simulink model "sampleModel2432_pp"  (R2018a)
settings: Solver=VariableStepAuto  StartTime=0.0  StopTime=10.0  RelTol=1e-3
undefined symbols (not defined in the file or in its folder): DiscIntNeverNeededParam, sigbuilder_block
libraries: simulink x354
(part 4 of 8)

== system sampleModel2432_pp/cfblk235 ==
  cfblk1 : Inport
  Action Port : ActionPort  ActionType=then
  cfblk10 : Delay
  cfblk3 : Delay  ShowEnablePort=on
      settings: InputPortMap=u0,e6
  cfblk4 : DiscreteIntegrator  SampleTime=-1  ICPrevOutput=DiscIntNeverNeededParam  ICPrevScaledInput=DiscIntNeverNeededParam
  cfblk5 : simulink/Continuous/PID Controller  Controller=PID  TimeDomain=Discrete-time  SampleTime=-1  IntegratorMethod=Forward Euler  FilterMethod=Forward Euler  Form=Parallel  UseFilter=on  ControllerParametersSource=internal  P=1  I=1  D=0  N=100  InitialConditionSource=internal  InitialConditionForIntegrator=0  InitialConditionForFilter=0  ExternalReset=none  LimitOutput=off  UpperSaturationLimit=inf  LowerSaturationLimit=-inf  LinearizeAsGain=off  AntiWindupMode=none  Kb=1  TrackingMode=off  Kt=1  PParamMin=[]  PParamMax=[]  IParamMin=[]  IParamMax=[]  DParamMin=[]  DParamMax=[]  NParamMin=[]  NParamMax=[]  KbParamMin=[]  KbParamMax=[]  KtParamMin=[]  KtParamMax=[]  POutMin=[]  POutMax=[]  IOutMin=[]  IOutMax=[]  DOutMin=[]  DOutMax=[]  NOutMin=[]  NOutMax=[]  KbOutMin=[]  KbOutMax=[]  KtOutMin=[]  KtOutMax=[]  IntegratorOutMin=[]  IntegratorOutMax=[]  FilterOutMin=[]  FilterOutMax=[]  SumOutMin=[]  SumOutMax=[]  SumI1OutMin=[]  SumI1OutMax=[]  SumI2OutMin=[]  SumI2OutMax=[]  SumI3OutMin=[]  SumI3OutMax=[]  SumDOutMin=[]  SumDOutMax=[]  SaturationOutMin=[]  SaturationOutMax=[]  IntegratorContinuousStateAttributes=''  IntegratorStateMustResolveToSignalObject=off  IntegratorRTWStateStorageClass=Auto  FilterContinuousStateAttributes=''  FilterStateMustResolveToSignalObject=off  FilterRTWStateStorageClass=Auto  DifferentiatorICPrevScaledInput=0  DifferentiatorOutMin=[]  DifferentiatorOutMax=[]  FilterDiffOutCoefMin=[]  FilterDiffOutCoefMax=[]  SumDenOutMin=[]  SumDenOutMax=[]  SumNumOutMin=[]  SumNumOutMax=[]  ReciprocalOutMin=[]  ReciprocalOutMax=[]  DivideOutMin=[]  DivideOutMax=[]  TunerSelectOption=Transfer Function Based (PID Tuner App)
  cfblk6 : Delay  ShowEnablePort=on
      settings: InputPortMap=u0,e6
  cfblk7 : Delay
  cfblk9 : Delay
  cyemi_{926..934} (9 alike) : DataTypeConversion  OutDataTypeStr=double
  cfblk2 : Outport
  cfblk8 : Outport  Port=2
  wires:
  cfblk1/1 -> cfblk2/1, cyemi_931/1
  cfblk7/1 -> cfblk8/1, cyemi_926/1, cyemi_932/1
  cyemi_926/1 -> cfblk10/1
  cyemi_927/1 -> cfblk3/1
  cfblk9/1 -> cyemi_927/1
  cyemi_928/1 -> cfblk3/2
  cfblk6/1 -> cyemi_928/1
  cyemi_929/1 -> cfblk4/1
  cfblk10/1 -> cyemi_929/1
  cyemi_930/1 -> cfblk5/1
  cfblk3/1 -> cyemi_930/1
  cyemi_931/1 -> cfblk6/1
  cyemi_932/1 -> cfblk6/2
  cyemi_933/1 -> cfblk7/1
  cfblk4/1 -> cyemi_933/1
  cyemi_934/1 -> cfblk9/1
  cfblk5/1 -> cyemi_934/1

== system sampleModel2432_pp/cfblk236 ==
  cfblk1 : Inport
  Action Port : ActionPort  ActionType=else
  cfblk{9..12} (4 alike) : DiscreteIntegrator  SampleTime=-1  ICPrevOutput=DiscIntNeverNeededParam  ICPrevScaledInput=DiscIntNeverNeededParam
  cfblk13 : simulink/Discrete/Transfer Fcn First Order  PoleZ=0.95  ICPrevOutput=0.0  DoSatur=off
      settings: SourceProductName=Simulink
  cfblk3 : simulink/Continuous/PID Controller  Controller=PID  TimeDomain=Discrete-time  SampleTime=-1  IntegratorMethod=Forward Euler  FilterMethod=Forward Euler  Form=Parallel  UseFilter=on  ControllerParametersSource=internal  P=1  I=1  D=0  N=100  InitialConditionSource=internal  InitialConditionForIntegrator=0  InitialConditionForFilter=0  ExternalReset=none  LimitOutput=off  UpperSaturationLimit=inf  LowerSaturationLimit=-inf  LinearizeAsGain=off  AntiWindupMode=none  Kb=1  TrackingMode=off  Kt=1  PParamMin=[]  PParamMax=[]  IParamMin=[]  IParamMax=[]  DParamMin=[]  DParamMax=[]  NParamMin=[]  NParamMax=[]  KbParamMin=[]  KbParamMax=[]  KtParamMin=[]  KtParamMax=[]  POutMin=[]  POutMax=[]  IOutMin=[]  IOutMax=[]  DOutMin=[]  DOutMax=[]  NOutMin=[]  NOutMax=[]  KbOutMin=[]  KbOutMax=[]  KtOutMin=[]  KtOutMax=[]  IntegratorOutMin=[]  IntegratorOutMax=[]  FilterOutMin=[]  FilterOutMax=[]  SumOutMin=[]  SumOutMax=[]  SumI1OutMin=[]  SumI1OutMax=[]  SumI2OutMin=[]  SumI2OutMax=[]  SumI3OutMin=[]  SumI3OutMax=[]  SumDOutMin=[]  SumDOutMax=[]  SaturationOutMin=[]  SaturationOutMax=[]  IntegratorContinuousStateAttributes=''  IntegratorStateMustResolveToSignalObject=off  IntegratorRTWStateStorageClass=Auto  FilterContinuousStateAttributes=''  FilterStateMustResolveToSignalObject=off  FilterRTWStateStorageClass=Auto  DifferentiatorICPrevScaledInput=0  DifferentiatorOutMin=[]  DifferentiatorOutMax=[]  FilterDiffOutCoefMin=[]  FilterDiffOutCoefMax=[]  SumDenOutMin=[]  SumDenOutMax=[]  SumNumOutMin=[]  SumNumOutMax=[]  ReciprocalOutMin=[]  ReciprocalOutMax=[]  DivideOutMin=[]  DivideOutMax=[]  TunerSelectOption=Transfer Function Based (PID Tuner App)
  cfblk4 : simulink/Discrete/Tapped Delay  vinit=0.0  samptime=-1  NumDelays=1  DelayOrder=Oldest  includeCurrent=off
  cfblk5 : Delay  DelayLengthSource=Input port
      settings: InputPortMap=u0,p1
  cfblk6 : Delay  ShowEnablePort=on
      settings: InputPortMap=u0,e6
  cfblk7 : Delay
  cfblk8 : DiscreteTransferFcn
  cyemi_{936..948} (13 alike) : DataTypeConversion  OutDataTypeStr=double
  cfblk2 : Outport
  wires:
  cfblk3/1 -> cyemi_939/1, cyemi_941/1
  cfblk1/1 -> cyemi_940/1, cyemi_945/1
  cfblk5/1 -> cfblk2/1
  cyemi_936/1 -> cfblk10/1
  cfblk8/1 -> cyemi_936/1
  cyemi_937/1 -> cfblk11/1
  cfblk12/1 -> cyemi_937/1
  cyemi_938/1 -> cfblk12/1
  cfblk10/1 -> cyemi_938/1
  cyemi_939/1 -> cfblk13/1
  cyemi_940/1 -> cfblk3/1
  cyemi_941/1 -> cfblk4/1
  cyemi_942/1 -> cfblk5/1
  cfblk7/1 -> cyemi_942/1
  cyemi_943/1 -> cfblk5/2
  cfblk11/1 -> cyemi_943/1
  cyemi_944/1 -> cfblk6/1
  cfblk4/1 -> cyemi_944/1
  cyemi_945/1 -> cfblk6/2
  cyemi_946/1 -> cfblk7/1
  cfblk6/1 -> cyemi_946/1
  cyemi_947/1 -> cfblk8/1
  cfblk9/1 -> cyemi_947/1
  cyemi_948/1 -> cfblk9/1
  cfblk13/1 -> cyemi_948/1

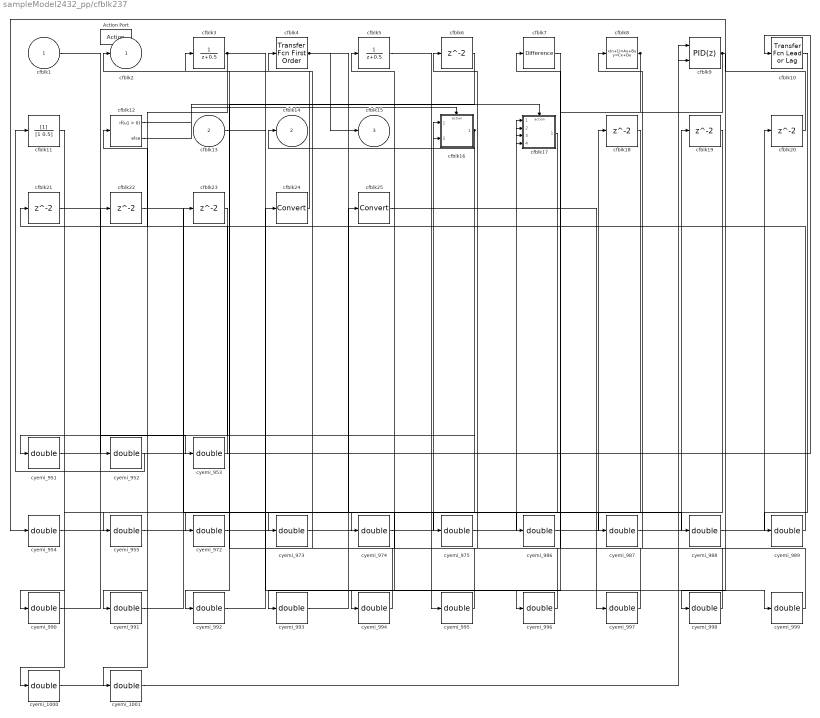
== system sampleModel2432_pp/cfblk237 ==
  cfblk1 : Inport
  cfblk13 : Inport  Port=2
  Action Port : ActionPort  ActionType=then
  cfblk10 : simulink/Discrete/Transfer Fcn Lead or Lag  PoleZ=0.95  ZeroZ=0.75  ICPrevOutput=0.0  ICPrevInput=0.0  DoSatur=off
      settings: SourceProductName=Simulink  SourceProductBaseCode=SL
  cfblk11 : DiscreteFilter
  cfblk12 : If  SampleTime=1
  cfblk16 : Subsystem  TreatAsAtomicUnit=on
  cfblk17 : Subsystem  TreatAsAtomicUnit=on
  cfblk{6,18..23} (7 alike) : Delay
  cfblk24 : DataTypeConversion
  cfblk25 : DataTypeConversion
  cfblk3 : DiscreteTransferFcn
  cfblk4 : simulink/Discrete/Transfer Fcn First Order  PoleZ=0.95  ICPrevOutput=0.0  DoSatur=off
      settings: SourceProductName=Simulink
  cfblk5 : DiscreteTransferFcn
  cfblk7 : simulink/Discrete/Difference  ICPrevInput=0.0  OutMin=[]  OutMax=[]  OutDataTypeStr=Inherit: Inherit via back propagation  OutDataType=fixdt(1, 16)  OutScaling=2^-10  DoSatur=off
  cfblk8 : DiscreteStateSpace  SampleTime=-1
  cfblk9 : simulink/Continuous/PID Controller (2DOF)  Controller=PID  TimeDomain=Discrete-time  SampleTime=-1  IntegratorMethod=Forward Euler  FilterMethod=Forward Euler  Form=Parallel  UseFilter=on  ControllerParametersSource=internal  P=1  I=1  D=0  N=100  b=1  c=1  InitialConditionSource=internal  InitialConditionForIntegrator=0  InitialConditionForFilter=0  ExternalReset=none  LimitOutput=off  UpperSaturationLimit=inf  LowerSaturationLimit=-inf  LinearizeAsGain=off  AntiWindupMode=none  Kb=1  TrackingMode=off  Kt=1  PParamMin=[]  PParamMax=[]  IParamMin=[]  IParamMax=[]  DParamMin=[]  DParamMax=[]  NParamMin=[]  NParamMax=[]  bParamMin=[]  bParamMax=[]  cParamMin=[]  cParamMax=[]  KbParamMin=[]  KbParamMax=[]  KtParamMin=[]  KtParamMax=[]  POutMin=[]  POutMax=[]  IOutMin=[]  IOutMax=[]  DOutMin=[]  DOutMax=[]  NOutMin=[]  NOutMax=[]  bOutMin=[]  bOutMax=[]  cOutMin=[]  cOutMax=[]  KbOutMin=[]  KbOutMax=[]  KtOutMin=[]  KtOutMax=[]  IntegratorOutMin=[]  IntegratorOutMax=[]  FilterOutMin=[]  FilterOutMax=[]  SumOutMin=[]  SumOutMax=[]  Sum1OutMin=[]  Sum1OutMax=[]  Sum2OutMin=[]  Sum2OutMax=[]  Sum3OutMin=[]  Sum3OutMax=[]  SumI1OutMin=[]  SumI1OutMax=[]  SumI2OutMin=[]  SumI2OutMax=[]  SumI3OutMin=[]  SumI3OutMax=[]  SumDOutMin=[]  SumDOutMax=[]  SaturationOutMin=[]  SaturationOutMax=[]  IntegratorContinuousStateAttributes=''  IntegratorStateMustResolveToSignalObject=off  IntegratorRTWStateStorageClass=Auto  FilterContinuousStateAttributes=''  FilterStateMustResolveToSignalObject=off  FilterRTWStateStorageClass=Auto  DifferentiatorICPrevScaledInput=0  DifferentiatorOutMin=[]  DifferentiatorOutMax=[]  FilterDiffOutCoefMin=[]  FilterDiffOutCoefMax=[]  SumDenOutMin=[]  SumDenOutMax=[]  SumNumOutMin=[]  SumNumOutMax=[]  ReciprocalOutMin=[]  ReciprocalOutMax=[]  DivideOutMin=[]  DivideOutMax=[]  TunerSelectOption=Transfer Function Based (PID Tuner App)
  cyemi_{951..955,972..975,986..1001} (25 alike) : DataTypeConversion  OutDataTypeStr=double
  cfblk2 : Outport
  cfblk14 : Outport  Port=2
  cfblk15 : Outport  Port=3
  wires:
  cfblk4/1 -> cfblk15/1, cyemi_986/1
  cfblk16/1(cfblk2) -> cfblk14/1, cyemi_951/1, cyemi_990/1
  cfblk8/1 -> cyemi_973/1, cyemi_993/1
  cfblk9/1 -> cyemi_975/1, cyemi_998/1
  cfblk3/1 -> cyemi_987/1, cyemi_988/1, cyemi_991/1
  cfblk12/1 -> cfblk16/Action
  cfblk12/2 -> cfblk17/Action
  cfblk24/1 -> cfblk2/1
  cyemi_951/1 -> cfblk10/1
  cyemi_952/1 -> cfblk11/1
  cfblk1/1 -> cyemi_952/1
  cyemi_953/1 -> cfblk12/1
  cfblk21/1 -> cyemi_953/1
  cyemi_954/1 -> cfblk16/1(cfblk1)
  cfblk20/1 -> cyemi_954/1
  cyemi_955/1 -> cfblk16/2(cfblk16)
  cfblk23/1 -> cyemi_955/1
  cyemi_972/1 -> cfblk17/1(cfblk1)
  cfblk19/1 -> cyemi_972/1
  cyemi_973/1 -> cfblk17/2(cfblk10)
  cyemi_974/1 -> cfblk17/3(cfblk11)
  cfblk22/1 -> cyemi_974/1
  cyemi_975/1 -> cfblk17/4(cfblk12)
  cyemi_986/1 -> cfblk18/1
  cyemi_987/1 -> cfblk19/1
  cyemi_988/1 -> cfblk20/1
  cyemi_989/1 -> cfblk21/1
  cfblk10/1 -> cyemi_989/1
  cyemi_990/1 -> cfblk22/1
  cyemi_991/1 -> cfblk23/1
  cyemi_992/1 -> cfblk24/1
  cfblk6/1 -> cyemi_992/1
  cyemi_993/1 -> cfblk25/1
  cyemi_994/1 -> cfblk3/1
  cfblk17/1(cfblk2) -> cyemi_994/1
  cyemi_995/1 -> cfblk4/1
  cfblk5/1 -> cyemi_995/1
  cyemi_996/1 -> cfblk5/1
  cfblk7/1 -> cyemi_996/1
  cyemi_997/1 -> cfblk6/1
  cfblk25/1 -> cyemi_997/1
  cyemi_998/1 -> cfblk7/1
  cyemi_999/1 -> cfblk8/1
  cfblk13/1 -> cyemi_999/1
  cyemi_1000/1 -> cfblk9/1
  cfblk11/1 -> cyemi_1000/1
  cyemi_1001/1 -> cfblk9/2
  cfblk18/1 -> cyemi_1001/1

== system sampleModel2432_pp/cfblk238 ==
  cfblk1 : Inport
  cfblk12 : Inport  Port=2
  Action Port : ActionPort  ActionType=else
  cfblk10 : DiscreteIntegrator  SampleTime=-1  ICPrevOutput=DiscIntNeverNeededParam  ICPrevScaledInput=DiscIntNeverNeededParam
  cfblk11 : Delay  ShowEnablePort=on
      settings: InputPortMap=u0,e6
  cfblk16 : Delay
  cfblk17 : Delay
  cfblk3 : DiscreteFilter
  cfblk4 : simulink/Discrete/Difference  ICPrevInput=0.0  OutMin=[]  OutMax=[]  OutDataTypeStr=Inherit: Inherit via back propagation  OutDataType=fixdt(1, 16)  OutScaling=2^-10  DoSatur=off
  cfblk5 : simulink/Continuous/PID Controller  Controller=PID  TimeDomain=Discrete-time  SampleTime=-1  IntegratorMethod=Forward Euler  FilterMethod=Forward Euler  Form=Parallel  UseFilter=on  ControllerParametersSource=internal  P=1  I=1  D=0  N=100  InitialConditionSource=internal  InitialConditionForIntegrator=0  InitialConditionForFilter=0  ExternalReset=none  LimitOutput=off  UpperSaturationLimit=inf  LowerSaturationLimit=-inf  LinearizeAsGain=off  AntiWindupMode=none  Kb=1  TrackingMode=off  Kt=1  PParamMin=[]  PParamMax=[]  IParamMin=[]  IParamMax=[]  DParamMin=[]  DParamMax=[]  NParamMin=[]  NParamMax=[]  KbParamMin=[]  KbParamMax=[]  KtParamMin=[]  KtParamMax=[]  POutMin=[]  POutMax=[]  IOutMin=[]  IOutMax=[]  DOutMin=[]  DOutMax=[]  NOutMin=[]  NOutMax=[]  KbOutMin=[]  KbOutMax=[]  KtOutMin=[]  KtOutMax=[]  IntegratorOutMin=[]  IntegratorOutMax=[]  FilterOutMin=[]  FilterOutMax=[]  SumOutMin=[]  SumOutMax=[]  SumI1OutMin=[]  SumI1OutMax=[]  SumI2OutMin=[]  SumI2OutMax=[]  SumI3OutMin=[]  SumI3OutMax=[]  SumDOutMin=[]  SumDOutMax=[]  SaturationOutMin=[]  SaturationOutMax=[]  IntegratorContinuousStateAttributes=''  IntegratorStateMustResolveToSignalObject=off  IntegratorRTWStateStorageClass=Auto  FilterContinuousStateAttributes=''  FilterStateMustResolveToSignalObject=off  FilterRTWStateStorageClass=Auto  DifferentiatorICPrevScaledInput=0  DifferentiatorOutMin=[]  DifferentiatorOutMax=[]  FilterDiffOutCoefMin=[]  FilterDiffOutCoefMax=[]  SumDenOutMin=[]  SumDenOutMax=[]  SumNumOutMin=[]  SumNumOutMax=[]  ReciprocalOutMin=[]  ReciprocalOutMax=[]  DivideOutMin=[]  DivideOutMax=[]  TunerSelectOption=Transfer Function Based (PID Tuner App)
  cfblk6 : simulink/Continuous/PID Controller (2DOF)  Controller=PID  TimeDomain=Discrete-time  SampleTime=-1  IntegratorMethod=Forward Euler  FilterMethod=Forward Euler  Form=Parallel  UseFilter=on  ControllerParametersSource=internal  P=1  I=1  D=0  N=100  b=1  c=1  InitialConditionSource=internal  InitialConditionForIntegrator=0  InitialConditionForFilter=0  ExternalReset=none  LimitOutput=off  UpperSaturationLimit=inf  LowerSaturationLimit=-inf  LinearizeAsGain=off  AntiWindupMode=none  Kb=1  TrackingMode=off  Kt=1  PParamMin=[]  PParamMax=[]  IParamMin=[]  IParamMax=[]  DParamMin=[]  DParamMax=[]  NParamMin=[]  NParamMax=[]  bParamMin=[]  bParamMax=[]  cParamMin=[]  cParamMax=[]  KbParamMin=[]  KbParamMax=[]  KtParamMin=[]  KtParamMax=[]  POutMin=[]  POutMax=[]  IOutMin=[]  IOutMax=[]  DOutMin=[]  DOutMax=[]  NOutMin=[]  NOutMax=[]  bOutMin=[]  bOutMax=[]  cOutMin=[]  cOutMax=[]  KbOutMin=[]  KbOutMax=[]  KtOutMin=[]  KtOutMax=[]  IntegratorOutMin=[]  IntegratorOutMax=[]  FilterOutMin=[]  FilterOutMax=[]  SumOutMin=[]  SumOutMax=[]  Sum1OutMin=[]  Sum1OutMax=[]  Sum2OutMin=[]  Sum2OutMax=[]  Sum3OutMin=[]  Sum3OutMax=[]  SumI1OutMin=[]  SumI1OutMax=[]  SumI2OutMin=[]  SumI2OutMax=[]  SumI3OutMin=[]  SumI3OutMax=[]  SumDOutMin=[]  SumDOutMax=[]  SaturationOutMin=[]  SaturationOutMax=[]  IntegratorContinuousStateAttributes=''  IntegratorStateMustResolveToSignalObject=off  IntegratorRTWStateStorageClass=Auto  FilterContinuousStateAttributes=''  FilterStateMustResolveToSignalObject=off  FilterRTWStateStorageClass=Auto  DifferentiatorICPrevScaledInput=0  DifferentiatorOutMin=[]  DifferentiatorOutMax=[]  FilterDiffOutCoefMin=[]  FilterDiffOutCoefMax=[]  SumDenOutMin=[]  SumDenOutMax=[]  SumNumOutMin=[]  SumNumOutMax=[]  ReciprocalOutMin=[]  ReciprocalOutMax=[]  DivideOutMin=[]  DivideOutMax=[]  TunerSelectOption=Transfer Function Based (PID Tuner App)
  cfblk7 : simulink/Discrete/Transfer Fcn First Order  PoleZ=0.95  ICPrevOutput=0.0  DoSatur=off
      settings: SourceProductName=Simulink
  cfblk8 : simulink/Discrete/Transfer Fcn First Order  PoleZ=0.95  ICPrevOutput=0.0  DoSatur=off
      settings: SourceProductName=Simulink
  cfblk9 : UnitDelay  SampleTime=-1
  cyemi_{1004..1016} (13 alike) : DataTypeConversion  OutDataTypeStr=double
  cfblk2 : Outport
  cfblk13 : Outport  Port=2
  cfblk14 : Outport  Port=3
  cfblk15 : Outport  Port=4
  wires:
  cfblk6/1 -> cfblk15/1, cyemi_1007/1
  cfblk9/1 -> cfblk14/1
  cfblk11/1 -> cyemi_1004/1, cyemi_1013/1, cyemi_1014/1
  cfblk3/1 -> cfblk2/1, cyemi_1010/1
  cfblk12/1 -> cfblk13/1
  cyemi_1004/1 -> cfblk10/1
  cyemi_1005/1 -> cfblk11/1
  cfblk5/1 -> cyemi_1005/1
  cyemi_1006/1 -> cfblk11/2
  cfblk16/1 -> cyemi_1006/1
  cyemi_1007/1 -> cfblk16/1
  cyemi_1008/1 -> cfblk17/1
  cfblk10/1 -> cyemi_1008/1
  cyemi_1009/1 -> cfblk3/1
  cfblk17/1 -> cyemi_1009/1
  cyemi_1010/1 -> cfblk4/1
  cyemi_1011/1 -> cfblk5/1
  cfblk4/1 -> cyemi_1011/1
  cyemi_1012/1 -> cfblk6/1
  cfblk7/1 -> cyemi_1012/1
  cyemi_1013/1 -> cfblk6/2
  cyemi_1014/1 -> cfblk7/1
  cyemi_1015/1 -> cfblk8/1
  cfblk1/1 -> cyemi_1015/1
  cyemi_1016/1 -> cfblk9/1
  cfblk8/1 -> cyemi_1016/1

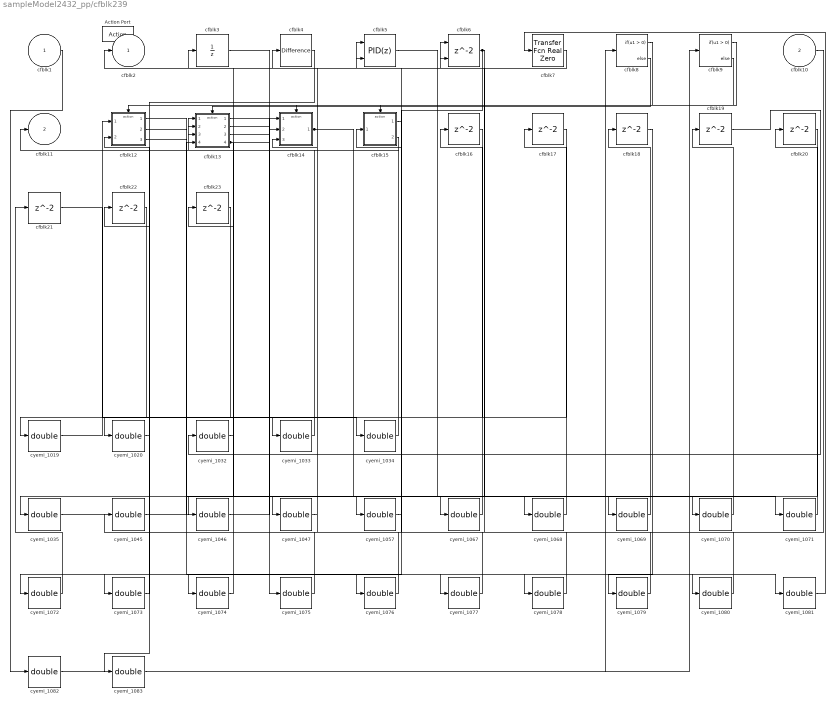
== system sampleModel2432_pp/cfblk239 ==
  cfblk1 : Inport
  cfblk10 : Inport  Port=2
  Action Port : ActionPort  ActionType=then
  cfblk12 : Subsystem  TreatAsAtomicUnit=on
  cfblk13 : Subsystem  TreatAsAtomicUnit=on
  cfblk14 : Subsystem  TreatAsAtomicUnit=on
  cfblk15 : Subsystem  TreatAsAtomicUnit=on
  cfblk{16..23} (8 alike) : Delay
  cfblk3 : UnitDelay  SampleTime=-1
  cfblk4 : simulink/Discrete/Difference  ICPrevInput=0.0  OutMin=[]  OutMax=[]  OutDataTypeStr=Inherit: Inherit via back propagation  OutDataType=fixdt(1, 16)  OutScaling=2^-10  DoSatur=off
  cfblk5 : simulink/Continuous/PID Controller (2DOF)  Controller=PID  TimeDomain=Discrete-time  SampleTime=-1  IntegratorMethod=Forward Euler  FilterMethod=Forward Euler  Form=Parallel  UseFilter=on  ControllerParametersSource=internal  P=1  I=1  D=0  N=100  b=1  c=1  InitialConditionSource=internal  InitialConditionForIntegrator=0  InitialConditionForFilter=0  ExternalReset=none  LimitOutput=off  UpperSaturationLimit=inf  LowerSaturationLimit=-inf  LinearizeAsGain=off  AntiWindupMode=none  Kb=1  TrackingMode=off  Kt=1  PParamMin=[]  PParamMax=[]  IParamMin=[]  IParamMax=[]  DParamMin=[]  DParamMax=[]  NParamMin=[]  NParamMax=[]  bParamMin=[]  bParamMax=[]  cParamMin=[]  cParamMax=[]  KbParamMin=[]  KbParamMax=[]  KtParamMin=[]  KtParamMax=[]  POutMin=[]  POutMax=[]  IOutMin=[]  IOutMax=[]  DOutMin=[]  DOutMax=[]  NOutMin=[]  NOutMax=[]  bOutMin=[]  bOutMax=[]  cOutMin=[]  cOutMax=[]  KbOutMin=[]  KbOutMax=[]  KtOutMin=[]  KtOutMax=[]  IntegratorOutMin=[]  IntegratorOutMax=[]  FilterOutMin=[]  FilterOutMax=[]  SumOutMin=[]  SumOutMax=[]  Sum1OutMin=[]  Sum1OutMax=[]  Sum2OutMin=[]  Sum2OutMax=[]  Sum3OutMin=[]  Sum3OutMax=[]  SumI1OutMin=[]  SumI1OutMax=[]  SumI2OutMin=[]  SumI2OutMax=[]  SumI3OutMin=[]  SumI3OutMax=[]  SumDOutMin=[]  SumDOutMax=[]  SaturationOutMin=[]  SaturationOutMax=[]  IntegratorContinuousStateAttributes=''  IntegratorStateMustResolveToSignalObject=off  IntegratorRTWStateStorageClass=Auto  FilterContinuousStateAttributes=''  FilterStateMustResolveToSignalObject=off  FilterRTWStateStorageClass=Auto  DifferentiatorICPrevScaledInput=0  DifferentiatorOutMin=[]  DifferentiatorOutMax=[]  FilterDiffOutCoefMin=[]  FilterDiffOutCoefMax=[]  SumDenOutMin=[]  SumDenOutMax=[]  SumNumOutMin=[]  SumNumOutMax=[]  ReciprocalOutMin=[]  ReciprocalOutMax=[]  DivideOutMin=[]  DivideOutMax=[]  TunerSelectOption=Transfer Function Based (PID Tuner App)
  cfblk6 : Delay  ShowEnablePort=on
      settings: InputPortMap=u0,e6
  cfblk7 : simulink/Discrete/Transfer Fcn Real Zero  ZeroZ=0.75  ICPrevInput=0.0  DoSatur=off
      settings: SourceProductName=Simulink  SourceProductBaseCode=SL
  cfblk8 : If  SampleTime=1
  cfblk9 : If  SampleTime=1
  cyemi_{1019..1020,1032..1035,1045..1047,1057,1067..1083} (27 alike) : DataTypeConversion  OutDataTypeStr=double
  cfblk2 : Outport
  cfblk11 : Outport  Port=2
  wires:
  cfblk7/1 -> cfblk2/1
  cfblk14/1(cfblk2) -> cyemi_1070/1, cyemi_1071/1
  cfblk15/2(cfblk11) -> cfblk11/1
  cfblk6/1 -> cyemi_1047/1, cyemi_1067/1, cyemi_1072/1
  cfblk13/4(cfblk16) -> cyemi_1046/1, cyemi_1081/1
  cfblk8/1 -> cfblk12/Action
  cfblk8/2 -> cfblk13/Action
  cfblk9/1 -> cfblk14/Action
  cfblk9/2 -> cfblk15/Action
  cyemi_1019/1 -> cfblk12/1(cfblk1)
  cfblk17/1 -> cyemi_1019/1
  cyemi_1020/1 -> cfblk12/2(cfblk12)
  cfblk22/1 -> cyemi_1020/1
  cyemi_1032/1 -> cfblk13/1(cfblk1)
  cfblk19/1 -> cyemi_1032/1
  cyemi_1033/1 -> cfblk13/2(cfblk11)
  cfblk16/1 -> cyemi_1033/1
  cyemi_1034/1 -> cfblk13/3(cfblk12)
  cfblk21/1 -> cyemi_1034/1
  cyemi_1035/1 -> cfblk13/4(cfblk13)
  cfblk20/1 -> cyemi_1035/1
  cyemi_1045/1 -> cfblk14/1(cfblk1)
  cfblk10/1 -> cyemi_1045/1
  cyemi_1046/1 -> cfblk14/2(cfblk12)
  cyemi_1047/1 -> cfblk14/3(cfblk13)
  cyemi_1057/1 -> cfblk15/1(cfblk1)
  cfblk12/3(cfblk14) -> cyemi_1057/1
  cyemi_1067/1 -> cfblk16/1
  cyemi_1068/1 -> cfblk17/1
  cfblk5/1 -> cyemi_1068/1
  cyemi_1069/1 -> cfblk18/1
  cfblk3/1 -> cyemi_1069/1
  cyemi_1070/1 -> cfblk19/1
  cyemi_1071/1 -> cfblk20/1
  cyemi_1072/1 -> cfblk21/1
  cyemi_1073/1 -> cfblk22/1
  cfblk4/1 -> cyemi_1073/1
  cyemi_1074/1 -> cfblk23/1
  cfblk15/1(cfblk2) -> cyemi_1074/1
  cyemi_1075/1 -> cfblk3/1
  cfblk13/3(cfblk15) -> cyemi_1075/1
  cyemi_1076/1 -> cfblk4/1
  cfblk12/2(cfblk13) -> cyemi_1076/1
  cyemi_1077/1 -> cfblk5/1
  cfblk13/1(cfblk2) -> cyemi_1077/1
  cyemi_1078/1 -> cfblk5/2
  cfblk13/2(cfblk14) -> cyemi_1078/1
  cyemi_1079/1 -> cfblk6/1
  cfblk18/1 -> cyemi_1079/1
  cyemi_1080/1 -> cfblk6/2
  cfblk12/1(cfblk2) -> cyemi_1080/1
  cyemi_1081/1 -> cfblk7/1
  cyemi_1082/1 -> cfblk8/1
  cfblk1/1 -> cyemi_1082/1
  cyemi_1083/1 -> cfblk9/1
  cfblk23/1 -> cyemi_1083/1

== system sampleModel2432_pp/cfblk240 ==
  cfblk1 : Inport
  cfblk7 : Inport  Port=2
  Action Port : ActionPort  ActionType=else
  cfblk3 : simulink/Discrete/Tapped Delay  vinit=0.0  samptime=-1  NumDelays=1  DelayOrder=Oldest  includeCurrent=off
  cfblk4 : DiscreteTransferFcn
  cfblk5 : simulink/Continuous/PID Controller  Controller=PID  TimeDomain=Discrete-time  SampleTime=-1  IntegratorMethod=Forward Euler  FilterMethod=Forward Euler  Form=Parallel  UseFilter=on  ControllerParametersSource=internal  P=1  I=1  D=0  N=100  InitialConditionSource=internal  InitialConditionForIntegrator=0  InitialConditionForFilter=0  ExternalReset=none  LimitOutput=off  UpperSaturationLimit=inf  LowerSaturationLimit=-inf  LinearizeAsGain=off  AntiWindupMode=none  Kb=1  TrackingMode=off  Kt=1  PParamMin=[]  PParamMax=[]  IParamMin=[]  IParamMax=[]  DParamMin=[]  DParamMax=[]  NParamMin=[]  NParamMax=[]  KbParamMin=[]  KbParamMax=[]  KtParamMin=[]  KtParamMax=[]  POutMin=[]  POutMax=[]  IOutMin=[]  IOutMax=[]  DOutMin=[]  DOutMax=[]  NOutMin=[]  NOutMax=[]  KbOutMin=[]  KbOutMax=[]  KtOutMin=[]  KtOutMax=[]  IntegratorOutMin=[]  IntegratorOutMax=[]  FilterOutMin=[]  FilterOutMax=[]  SumOutMin=[]  SumOutMax=[]  SumI1OutMin=[]  SumI1OutMax=[]  SumI2OutMin=[]  SumI2OutMax=[]  SumI3OutMin=[]  SumI3OutMax=[]  SumDOutMin=[]  SumDOutMax=[]  SaturationOutMin=[]  SaturationOutMax=[]  IntegratorContinuousStateAttributes=''  IntegratorStateMustResolveToSignalObject=off  IntegratorRTWStateStorageClass=Auto  FilterContinuousStateAttributes=''  FilterStateMustResolveToSignalObject=off  FilterRTWStateStorageClass=Auto  DifferentiatorICPrevScaledInput=0  DifferentiatorOutMin=[]  DifferentiatorOutMax=[]  FilterDiffOutCoefMin=[]  FilterDiffOutCoefMax=[]  SumDenOutMin=[]  SumDenOutMax=[]  SumNumOutMin=[]  SumNumOutMax=[]  ReciprocalOutMin=[]  ReciprocalOutMax=[]  DivideOutMin=[]  DivideOutMax=[]  TunerSelectOption=Transfer Function Based (PID Tuner App)
  cfblk6 : simulink/Continuous/PID Controller  Controller=PID  TimeDomain=Discrete-time  SampleTime=-1  IntegratorMethod=Forward Euler  FilterMethod=Forward Euler  Form=Parallel  UseFilter=on  ControllerParametersSource=internal  P=1  I=1  D=0  N=100  InitialConditionSource=internal  InitialConditionForIntegrator=0  InitialConditionForFilter=0  ExternalReset=none  LimitOutput=off  UpperSaturationLimit=inf  LowerSaturationLimit=-inf  LinearizeAsGain=off  AntiWindupMode=none  Kb=1  TrackingMode=off  Kt=1  PParamMin=[]  PParamMax=[]  IParamMin=[]  IParamMax=[]  DParamMin=[]  DParamMax=[]  NParamMin=[]  NParamMax=[]  KbParamMin=[]  KbParamMax=[]  KtParamMin=[]  KtParamMax=[]  POutMin=[]  POutMax=[]  IOutMin=[]  IOutMax=[]  DOutMin=[]  DOutMax=[]  NOutMin=[]  NOutMax=[]  KbOutMin=[]  KbOutMax=[]  KtOutMin=[]  KtOutMax=[]  IntegratorOutMin=[]  IntegratorOutMax=[]  FilterOutMin=[]  FilterOutMax=[]  SumOutMin=[]  SumOutMax=[]  SumI1OutMin=[]  SumI1OutMax=[]  SumI2OutMin=[]  SumI2OutMax=[]  SumI3OutMin=[]  SumI3OutMax=[]  SumDOutMin=[]  SumDOutMax=[]  SaturationOutMin=[]  SaturationOutMax=[]  IntegratorContinuousStateAttributes=''  IntegratorStateMustResolveToSignalObject=off  IntegratorRTWStateStorageClass=Auto  FilterContinuousStateAttributes=''  FilterStateMustResolveToSignalObject=off  FilterRTWStateStorageClass=Auto  DifferentiatorICPrevScaledInput=0  DifferentiatorOutMin=[]  DifferentiatorOutMax=[]  FilterDiffOutCoefMin=[]  FilterDiffOutCoefMax=[]  SumDenOutMin=[]  SumDenOutMax=[]  SumNumOutMin=[]  SumNumOutMax=[]  ReciprocalOutMin=[]  ReciprocalOutMax=[]  DivideOutMin=[]  DivideOutMax=[]  TunerSelectOption=Transfer Function Based (PID Tuner App)
  cfblk9 : Delay
  cyemi_{1087..1091} (5 alike) : DataTypeConversion  OutDataTypeStr=double
  cfblk2 : Outport
  cfblk8 : Outport  Port=2
  wires:
  cfblk6/1 -> cfblk2/1
  cfblk4/1 -> cfblk8/1
  cyemi_1087/1 -> cfblk3/1
  cfblk9/1 -> cyemi_1087/1
  cyemi_1088/1 -> cfblk4/1
  cfblk7/1 -> cyemi_1088/1
  cyemi_1089/1 -> cfblk5/1
  cfblk3/1 -> cyemi_1089/1
  cyemi_1090/1 -> cfblk6/1
  cfblk1/1 -> cyemi_1090/1
  cyemi_1091/1 -> cfblk9/1
  cfblk5/1 -> cyemi_1091/1

== system sampleModel2432_pp/cfblk241 ==
  cfblk1 : Inport
  cfblk8 : Inport  Port=2
  cfblk9 : Inport  Port=3
  cfblk10 : Inport  Port=4
  cfblk11 : Inport  Port=5
  Action Port : ActionPort  ActionType=then
  cfblk13 : Delay
  cfblk3 : Delay
  cfblk4 : Delay  ShowEnablePort=on
      settings: InputPortMap=u0,e6
  cfblk5 : UnitDelay  SampleTime=-1
  cfblk6 : Delay  ShowEnablePort=on
      settings: InputPortMap=u0,e6
  cfblk7 : DiscreteStateSpace  SampleTime=-1
  cyemi_{1097..1104} (8 alike) : DataTypeConversion  OutDataTypeStr=double
  cfblk2 : Outport
  cfblk12 : Outport  Port=2
  wires:
  cfblk9/1 -> cfblk2/1
  cfblk3/1 -> cfblk12/1
  cyemi_1097/1 -> cfblk13/1
  cfblk4/1 -> cyemi_1097/1
  cyemi_1098/1 -> cfblk3/1
  cfblk10/1 -> cyemi_1098/1
  cyemi_1099/1 -> cfblk4/1
  cfblk6/1 -> cyemi_1099/1
  cyemi_1100/1 -> cfblk4/2
  cfblk7/1 -> cyemi_1100/1
  cyemi_1101/1 -> cfblk5/1
  cfblk8/1 -> cyemi_1101/1
  cyemi_1102/1 -> cfblk6/1
  cfblk13/1 -> cyemi_1102/1
  cyemi_1103/1 -> cfblk6/2
  cfblk1/1 -> cyemi_1103/1
  cyemi_1104/1 -> cfblk7/1
  cfblk5/1 -> cyemi_1104/1

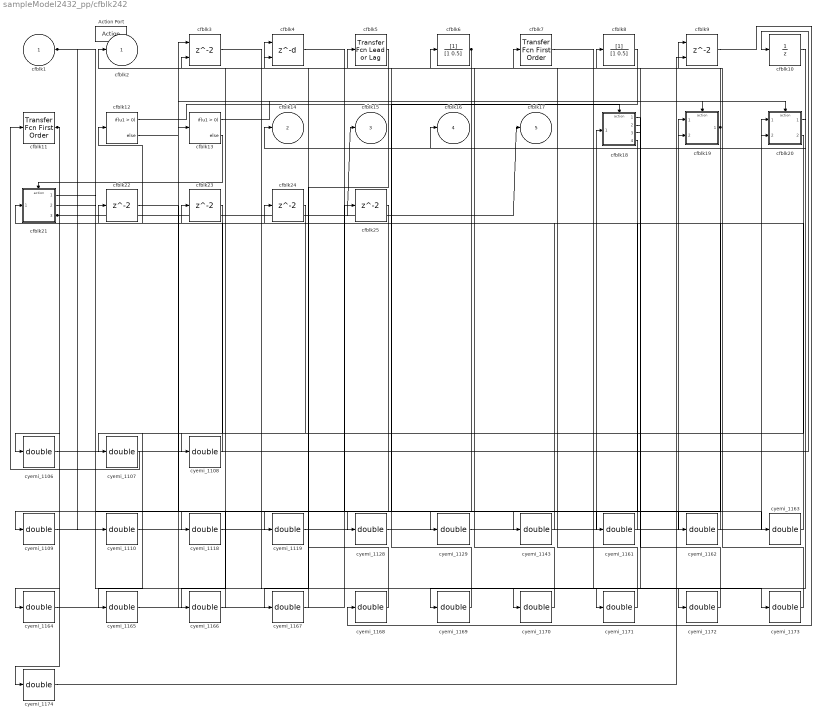
== system sampleModel2432_pp/cfblk242 ==
  cfblk1 : Inport
  Action Port : ActionPort  ActionType=else
  cfblk10 : UnitDelay  SampleTime=-1
  cfblk11 : simulink/Discrete/Transfer Fcn First Order  PoleZ=0.95  ICPrevOutput=0.0  DoSatur=off
      settings: SourceProductName=Simulink
  cfblk12 : If  SampleTime=1
  cfblk13 : If  SampleTime=1
  cfblk18 : Subsystem  TreatAsAtomicUnit=on
  cfblk19 : Subsystem  TreatAsAtomicUnit=on
  cfblk20 : Subsystem  TreatAsAtomicUnit=on
  cfblk21 : Subsystem  TreatAsAtomicUnit=on
  cfblk{22..25} (4 alike) : Delay
  cfblk3 : Delay  ShowEnablePort=on
      settings: InputPortMap=u0,e6
  cfblk4 : Delay  DelayLengthSource=Input port
      settings: InputPortMap=u0,p1
  cfblk5 : simulink/Discrete/Transfer Fcn Lead or Lag  PoleZ=0.95  ZeroZ=0.75  ICPrevOutput=0.0  ICPrevInput=0.0  DoSatur=off
      settings: SourceProductName=Simulink  SourceProductBaseCode=SL
  cfblk6 : DiscreteFilter
  cfblk7 : simulink/Discrete/Transfer Fcn First Order  PoleZ=0.95  ICPrevOutput=0.0  DoSatur=off
      settings: SourceProductName=Simulink
  cfblk8 : DiscreteFilter
  cfblk9 : Delay  ShowEnablePort=on
      settings: InputPortMap=u0,e6
  cyemi_{1106..1110,1118..1119,1128..1129,1143,1161..1174} (24 alike) : DataTypeConversion  OutDataTypeStr=double
  cfblk2 : Outport
  cfblk14 : Outport  Port=2
  cfblk15 : Outport  Port=3
  cfblk16 : Outport  Port=4
  cfblk17 : Outport  Port=5
  wires:
  cfblk1/1 -> cyemi_1110/1, cyemi_1170/1
  cfblk10/1 -> cfblk16/1
  cfblk19/1(cfblk2) -> cfblk2/1, cyemi_1166/1
  cfblk6/1 -> cyemi_1119/1, cyemi_1174/1
  cfblk18/3(cfblk10) -> cfblk14/1
  cfblk11/1 -> cyemi_1106/1, cyemi_1164/1
  cfblk21/3(cfblk16) -> cfblk15/1, cfblk17/1
  cfblk12/1 -> cfblk18/Action
  cfblk12/2 -> cfblk19/Action
  cfblk13/1 -> cfblk20/Action
  cfblk13/2 -> cfblk21/Action
  cyemi_1106/1 -> cfblk10/1
  cyemi_1107/1 -> cfblk11/1
  cfblk20/2(cfblk14) -> cyemi_1107/1
  cyemi_1108/1 -> cfblk12/1
  cfblk24/1 -> cyemi_1108/1
  cyemi_1109/1 -> cfblk13/1
  cfblk25/1 -> cyemi_1109/1
  cyemi_1110/1 -> cfblk18/1(cfblk1)
  cyemi_1118/1 -> cfblk19/1(cfblk1)
  cfblk18/1(cfblk2) -> cyemi_1118/1
  cyemi_1119/1 -> cfblk19/2(cfblk10)
  cyemi_1128/1 -> cfblk20/1(cfblk1)
  cfblk8/1 -> cyemi_1128/1
  cyemi_1129/1 -> cfblk20/2(cfblk13)
  cfblk18/4(cfblk11) -> cyemi_1129/1
  cyemi_1143/1 -> cfblk21/1(cfblk1)
  cfblk22/1 -> cyemi_1143/1
  cyemi_1161/1 -> cfblk22/1
  cfblk4/1 -> cyemi_1161/1
  cyemi_1162/1 -> cfblk23/1
  cfblk21/1(cfblk2) -> cyemi_1162/1
  cyemi_1163/1 -> cfblk24/1
  cfblk21/2(cfblk15) -> cyemi_1163/1
  cyemi_1164/1 -> cfblk25/1
  cyemi_1165/1 -> cfblk3/1
  cfblk23/1 -> cyemi_1165/1
  cyemi_1166/1 -> cfblk3/2
  cyemi_1167/1 -> cfblk4/1
  cfblk5/1 -> cyemi_1167/1
  cyemi_1168/1 -> cfblk4/2
  cfblk9/1 -> cyemi_1168/1
  cyemi_1169/1 -> cfblk5/1
  cfblk20/1(cfblk2) -> cyemi_1169/1
  cyemi_1170/1 -> cfblk6/1
  cyemi_1171/1 -> cfblk7/1
  cfblk18/2(cfblk9) -> cyemi_1171/1
  cyemi_1172/1 -> cfblk8/1
  cfblk3/1 -> cyemi_1172/1
  cyemi_1173/1 -> cfblk9/1
  cfblk7/1 -> cyemi_1173/1
  cyemi_1174/1 -> cfblk9/2

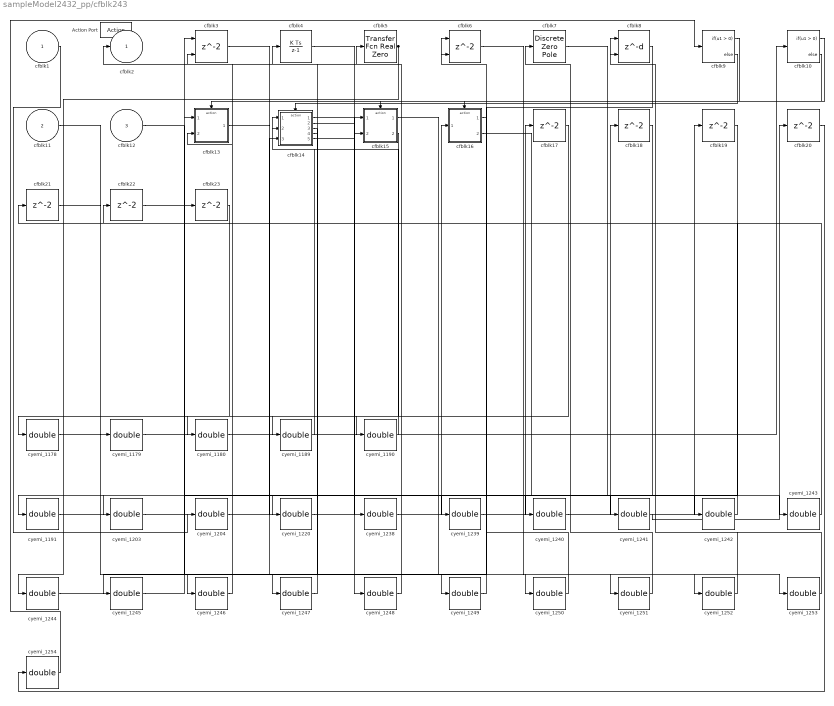
== system sampleModel2432_pp/cfblk243 ==
  cfblk1 : Inport
  cfblk11 : Inport  Port=2
  cfblk12 : Inport  Port=3
  Action Port : ActionPort  ActionType=then
  cfblk10 : If  SampleTime=1
  cfblk13 : Subsystem  TreatAsAtomicUnit=on
  cfblk14 : Subsystem  TreatAsAtomicUnit=on
  cfblk15 : Subsystem  TreatAsAtomicUnit=on
  cfblk16 : Subsystem  TreatAsAtomicUnit=on
  cfblk{17..23} (7 alike) : Delay
  cfblk3 : Delay  ShowEnablePort=on
      settings: InputPortMap=u0,e6
  cfblk4 : DiscreteIntegrator  SampleTime=-1  ICPrevOutput=DiscIntNeverNeededParam  ICPrevScaledInput=DiscIntNeverNeededParam
  cfblk5 : simulink/Discrete/Transfer Fcn Real Zero  ZeroZ=0.75  ICPrevInput=0.0  DoSatur=off
      settings: SourceProductName=Simulink  SourceProductBaseCode=SL
  cfblk6 : Delay  ShowEnablePort=on
      settings: InputPortMap=u0,e6
  cfblk7 : DiscreteZeroPole  Poles=[0 0.5]  Gain=1  SampleTime=-1
  cfblk8 : Delay  DelayLengthSource=Input port
      settings: InputPortMap=u0,p1
  cfblk9 : If  SampleTime=1
  cyemi_{1178..1180,1189..1191,1203..1204,1220,1238..1254} (26 alike) : DataTypeConversion  OutDataTypeStr=double
  cfblk2 : Outport
  wires:
  cfblk5/1 -> cfblk2/1, cyemi_1244/1
  cfblk9/1 -> cfblk13/Action
  cfblk9/2 -> cfblk14/Action
  cfblk10/1 -> cfblk15/Action
  cfblk10/2 -> cfblk16/Action
  cyemi_1178/1 -> cfblk10/1
  cfblk17/1 -> cyemi_1178/1
  cyemi_1179/1 -> cfblk13/1(cfblk1)
  cfblk11/1 -> cyemi_1179/1
  cyemi_1180/1 -> cfblk13/2(cfblk10)
  cfblk23/1 -> cyemi_1180/1
  cyemi_1189/1 -> cfblk14/1(cfblk1)
  cfblk8/1 -> cyemi_1189/1
  cyemi_1190/1 -> cfblk14/2(cfblk11)
  cfblk15/2(cfblk16) -> cyemi_1190/1
  cyemi_1191/1 -> cfblk14/3(cfblk12)
  cfblk18/1 -> cyemi_1191/1
  cyemi_1203/1 -> cfblk15/1(cfblk1)
  cfblk19/1 -> cyemi_1203/1
  cyemi_1204/1 -> cfblk15/2(cfblk15)
  cfblk1/1 -> cyemi_1204/1
  cyemi_1220/1 -> cfblk16/1(cfblk1)
  cfblk12/1 -> cyemi_1220/1
  cyemi_1238/1 -> cfblk17/1
  cfblk14/1(cfblk2) -> cyemi_1238/1
  cyemi_1239/1 -> cfblk18/1
  cfblk4/1 -> cyemi_1239/1
  cyemi_1240/1 -> cfblk19/1
  cfblk13/1(cfblk2) -> cyemi_1240/1
  cyemi_1241/1 -> cfblk20/1
  cfblk16/2(cfblk14) -> cyemi_1241/1
  cyemi_1242/1 -> cfblk21/1
  cfblk14/2(cfblk13) -> cyemi_1242/1
  cyemi_1243/1 -> cfblk22/1
  cfblk7/1 -> cyemi_1243/1
  cyemi_1244/1 -> cfblk23/1
  cyemi_1245/1 -> cfblk3/1
  cfblk14/3(cfblk14) -> cyemi_1245/1
  cyemi_1246/1 -> cfblk3/2
  cfblk14/4(cfblk15) -> cyemi_1246/1
  cyemi_1247/1 -> cfblk4/1
  cfblk16/1(cfblk2) -> cyemi_1247/1
  cyemi_1248/1 -> cfblk5/1
  cfblk14/5(cfblk16) -> cyemi_1248/1
  cyemi_1249/1 -> cfblk6/1
  cfblk3/1 -> cyemi_1249/1
  cyemi_1250/1 -> cfblk6/2
  cfblk22/1 -> cyemi_1250/1
  cyemi_1251/1 -> cfblk7/1
  cfblk6/1 -> cyemi_1251/1
  cyemi_1252/1 -> cfblk8/1
  cfblk15/1(cfblk2) -> cyemi_1252/1
  cyemi_1253/1 -> cfblk8/2
  cfblk21/1 -> cyemi_1253/1
  cyemi_1254/1 -> cfblk9/1
  cfblk20/1 -> cyemi_1254/1

== system sampleModel2432_pp/cfblk244 ==
  cfblk1 : Inport
  Action Port : ActionPort  ActionType=else
  cfblk10 : Subsystem  TreatAsAtomicUnit=on
  cfblk11 : Subsystem  TreatAsAtomicUnit=on
  cfblk{12..15} (4 alike) : Delay
  cfblk3 : simulink/Discrete/Transfer Fcn Lead or Lag  PoleZ=0.95  ZeroZ=0.75  ICPrevOutput=0.0  ICPrevInput=0.0  DoSatur=off
      settings: SourceProductName=Simulink  SourceProductBaseCode=SL
  cfblk4 : UnitDelay  SampleTime=-1
  cfblk5 : If  SampleTime=1
  cfblk6 : If  SampleTime=1
  cfblk8 : Subsystem  TreatAsAtomicUnit=on
  cfblk9 : Subsystem  TreatAsAtomicUnit=on
  cyemi_{1256,1262..1265,1273..1282,1287..1289} (18 alike) : DataTypeConversion  OutDataTypeStr=double
  cfblk2 : Outport
  cfblk7 : Outport  Port=2
  wires:
  cfblk3/1 -> cyemi_1273/1, cyemi_1289/1
  cfblk4/1 -> cfblk2/1, cyemi_1275/1, cyemi_1276/1, cyemi_1288/1
  cfblk10/2(cfblk7) -> cfblk7/1, cyemi_1278/1, cyemi_1279/1, cyemi_1281/1
  cfblk1/1 -> cyemi_1256/1, cyemi_1280/1
  cfblk5/1 -> cfblk8/Action
  cfblk5/2 -> cfblk9/Action
  cfblk6/1 -> cfblk10/Action
  cfblk6/2 -> cfblk11/Action
  cyemi_1256/1 -> cfblk10/1(cfblk1)
  cyemi_1262/1 -> cfblk11/1(cfblk1)
  cfblk13/1 -> cyemi_1262/1
  cyemi_1263/1 -> cfblk11/2(cfblk10)
  cfblk12/1 -> cyemi_1263/1
  cyemi_1264/1 -> cfblk11/3(cfblk11)
  cfblk14/1 -> cyemi_1264/1
  cyemi_1265/1 -> cfblk11/4(cfblk12)
  cfblk15/1 -> cyemi_1265/1
  cyemi_1273/1 -> cfblk12/1
  cyemi_1274/1 -> cfblk13/1
  cfblk8/1(cfblk2) -> cyemi_1274/1
  cyemi_1275/1 -> cfblk14/1
  cyemi_1276/1 -> cfblk15/1
  cyemi_1277/1 -> cfblk3/1
  cfblk10/1(cfblk2) -> cyemi_1277/1
  cyemi_1278/1 -> cfblk4/1
  cyemi_1279/1 -> cfblk5/1
  cyemi_1280/1 -> cfblk6/1
  cyemi_1281/1 -> cfblk8/1(cfblk1)
  cyemi_1282/1 -> cfblk8/2(cfblk7)
  cfblk9/1(cfblk2) -> cyemi_1282/1
  cyemi_1287/1 -> cfblk9/1(cfblk1)
  cfblk11/1(cfblk2) -> cyemi_1287/1
  cyemi_1288/1 -> cfblk9/2(cfblk8)
  cyemi_1289/1 -> cfblk9/3(cfblk9)

== system sampleModel2432_pp/cfblk196/cfblk12 ==
  cfblk1 : Inport
  cfblk10 : Inport  Port=2
  Action Port : ActionPort  ActionType=then
  cfblk3 : simulink/Discrete/Transfer Fcn First Order  PoleZ=0.95  ICPrevOutput=0.0  DoSatur=off
      settings: SourceProductName=Simulink
  cfblk4 : simulink/Discrete/Transfer Fcn First Order  PoleZ=0.95  ICPrevOutput=0.0  DoSatur=off
      settings: SourceProductName=Simulink
  cfblk5 : DiscreteFilter
  cfblk6 : Delay  ShowEnablePort=on
      settings: InputPortMap=u0,e6
  cfblk7 : simulink/Continuous/PID Controller (2DOF)  Controller=PID  TimeDomain=Discrete-time  SampleTime=-1  IntegratorMethod=Forward Euler  FilterMethod=Forward Euler  Form=Parallel  UseFilter=on  ControllerParametersSource=internal  P=1  I=1  D=0  N=100  b=1  c=1  InitialConditionSource=internal  InitialConditionForIntegrator=0  InitialConditionForFilter=0  ExternalReset=none  LimitOutput=off  UpperSaturationLimit=inf  LowerSaturationLimit=-inf  LinearizeAsGain=off  AntiWindupMode=none  Kb=1  TrackingMode=off  Kt=1  PParamMin=[]  PParamMax=[]  IParamMin=[]  IParamMax=[]  DParamMin=[]  DParamMax=[]  NParamMin=[]  NParamMax=[]  bParamMin=[]  bParamMax=[]  cParamMin=[]  cParamMax=[]  KbParamMin=[]  KbParamMax=[]  KtParamMin=[]  KtParamMax=[]  POutMin=[]  POutMax=[]  IOutMin=[]  IOutMax=[]  DOutMin=[]  DOutMax=[]  NOutMin=[]  NOutMax=[]  bOutMin=[]  bOutMax=[]  cOutMin=[]  cOutMax=[]  KbOutMin=[]  KbOutMax=[]  KtOutMin=[]  KtOutMax=[]  IntegratorOutMin=[]  IntegratorOutMax=[]  FilterOutMin=[]  FilterOutMax=[]  SumOutMin=[]  SumOutMax=[]  Sum1OutMin=[]  Sum1OutMax=[]  Sum2OutMin=[]  Sum2OutMax=[]  Sum3OutMin=[]  Sum3OutMax=[]  SumI1OutMin=[]  SumI1OutMax=[]  SumI2OutMin=[]  SumI2OutMax=[]  SumI3OutMin=[]  SumI3OutMax=[]  SumDOutMin=[]  SumDOutMax=[]  SaturationOutMin=[]  SaturationOutMax=[]  IntegratorContinuousStateAttributes=''  IntegratorStateMustResolveToSignalObject=off  IntegratorRTWStateStorageClass=Auto  FilterContinuousStateAttributes=''  FilterStateMustResolveToSignalObject=off  FilterRTWStateStorageClass=Auto  DifferentiatorICPrevScaledInput=0  DifferentiatorOutMin=[]  DifferentiatorOutMax=[]  FilterDiffOutCoefMin=[]  FilterDiffOutCoefMax=[]  SumDenOutMin=[]  SumDenOutMax=[]  SumNumOutMin=[]  SumNumOutMax=[]  ReciprocalOutMin=[]  ReciprocalOutMax=[]  DivideOutMin=[]  DivideOutMax=[]  TunerSelectOption=Transfer Function Based (PID Tuner App)
  cfblk8 : UnitDelay  SampleTime=-1
  cfblk9 : UnitDelay  SampleTime=-1
  cyemi_{60..68} (9 alike) : DataTypeConversion  OutDataTypeStr=double
  cfblk2 : Outport
  cfblk11 : Outport  Port=2
  cfblk12 : Outport  Port=3
  wires:
  cfblk5/1 -> cyemi_61/1, cyemi_66/1
  cfblk10/1 -> cfblk11/1
  cfblk4/1 -> cfblk2/1
  cfblk8/1 -> cyemi_63/1, cyemi_65/1, cyemi_68/1
  cfblk6/1 -> cfblk12/1
  cyemi_60/1 -> cfblk3/1
  cfblk9/1 -> cyemi_60/1
  cyemi_61/1 -> cfblk4/1
  cyemi_62/1 -> cfblk5/1
  cfblk3/1 -> cyemi_62/1
  cyemi_63/1 -> cfblk6/1
  cyemi_64/1 -> cfblk6/2
  cfblk7/1 -> cyemi_64/1
  cyemi_65/1 -> cfblk7/1
  cyemi_66/1 -> cfblk7/2
  cyemi_67/1 -> cfblk8/1
  cfblk1/1 -> cyemi_67/1
  cyemi_68/1 -> cfblk9/1

== system sampleModel2432_pp/cfblk196/cfblk13 ==
  cfblk1 : Inport
  cfblk8 : Inport  Port=2
  Action Port : ActionPort  ActionType=else
  cfblk3 : simulink/Discrete/Transfer Fcn Lead or Lag  PoleZ=0.95  ZeroZ=0.75  ICPrevOutput=0.0  ICPrevInput=0.0  DoSatur=off
      settings: SourceProductName=Simulink  SourceProductBaseCode=SL
  cfblk4 : UnitDelay  SampleTime=-1
  cfblk5 : Delay  DelayLengthSource=Input port
      settings: InputPortMap=u0,p1
  cfblk6 : DiscreteFir
  cfblk7 : simulink/Discrete/Tapped Delay  vinit=0.0  samptime=-1  NumDelays=1  DelayOrder=Oldest  includeCurrent=off
  cyemi_{71..76} (6 alike) : DataTypeConversion  OutDataTypeStr=double
  cfblk2 : Outport
  cfblk9 : Outport  Port=2
  wires:
  cfblk4/1 -> cyemi_75/1, cyemi_76/1
  cfblk3/1 -> cfblk9/1
  cfblk5/1 -> cfblk2/1
  cyemi_71/1 -> cfblk3/1
  cfblk6/1 -> cyemi_71/1
  cyemi_72/1 -> cfblk4/1
  cfblk1/1 -> cyemi_72/1
  cyemi_73/1 -> cfblk5/1
  cfblk8/1 -> cyemi_73/1
  cyemi_74/1 -> cfblk5/2
  cfblk7/1 -> cyemi_74/1
  cyemi_75/1 -> cfblk6/1
  cyemi_76/1 -> cfblk7/1

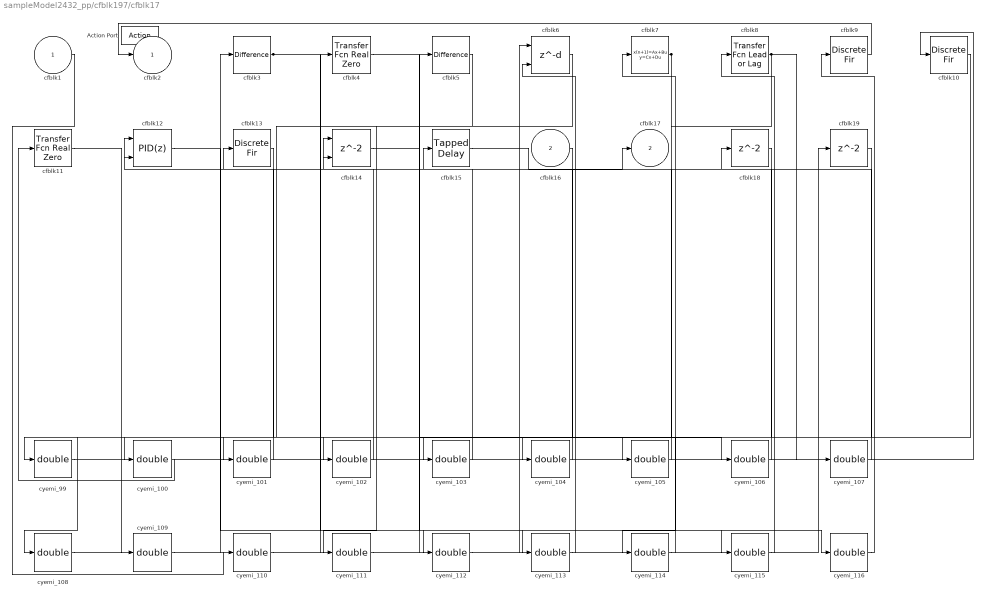
== system sampleModel2432_pp/cfblk197/cfblk17 ==
  cfblk1 : Inport
  cfblk16 : Inport  Port=2
  Action Port : ActionPort  ActionType=then
  cfblk10 : DiscreteFir
  cfblk11 : simulink/Discrete/Transfer Fcn Real Zero  ZeroZ=0.75  ICPrevInput=0.0  DoSatur=off
      settings: SourceProductName=Simulink  SourceProductBaseCode=SL
  cfblk12 : simulink/Continuous/PID Controller (2DOF)  Controller=PID  TimeDomain=Discrete-time  SampleTime=-1  IntegratorMethod=Forward Euler  FilterMethod=Forward Euler  Form=Parallel  UseFilter=on  ControllerParametersSource=internal  P=1  I=1  D=0  N=100  b=1  c=1  InitialConditionSource=internal  InitialConditionForIntegrator=0  InitialConditionForFilter=0  ExternalReset=none  LimitOutput=off  UpperSaturationLimit=inf  LowerSaturationLimit=-inf  LinearizeAsGain=off  AntiWindupMode=none  Kb=1  TrackingMode=off  Kt=1  PParamMin=[]  PParamMax=[]  IParamMin=[]  IParamMax=[]  DParamMin=[]  DParamMax=[]  NParamMin=[]  NParamMax=[]  bParamMin=[]  bParamMax=[]  cParamMin=[]  cParamMax=[]  KbParamMin=[]  KbParamMax=[]  KtParamMin=[]  KtParamMax=[]  POutMin=[]  POutMax=[]  IOutMin=[]  IOutMax=[]  DOutMin=[]  DOutMax=[]  NOutMin=[]  NOutMax=[]  bOutMin=[]  bOutMax=[]  cOutMin=[]  cOutMax=[]  KbOutMin=[]  KbOutMax=[]  KtOutMin=[]  KtOutMax=[]  IntegratorOutMin=[]  IntegratorOutMax=[]  FilterOutMin=[]  FilterOutMax=[]  SumOutMin=[]  SumOutMax=[]  Sum1OutMin=[]  Sum1OutMax=[]  Sum2OutMin=[]  Sum2OutMax=[]  Sum3OutMin=[]  Sum3OutMax=[]  SumI1OutMin=[]  SumI1OutMax=[]  SumI2OutMin=[]  SumI2OutMax=[]  SumI3OutMin=[]  SumI3OutMax=[]  SumDOutMin=[]  SumDOutMax=[]  SaturationOutMin=[]  SaturationOutMax=[]  IntegratorContinuousStateAttributes=''  IntegratorStateMustResolveToSignalObject=off  IntegratorRTWStateStorageClass=Auto  FilterContinuousStateAttributes=''  FilterStateMustResolveToSignalObject=off  FilterRTWStateStorageClass=Auto  DifferentiatorICPrevScaledInput=0  DifferentiatorOutMin=[]  DifferentiatorOutMax=[]  FilterDiffOutCoefMin=[]  FilterDiffOutCoefMax=[]  SumDenOutMin=[]  SumDenOutMax=[]  SumNumOutMin=[]  SumNumOutMax=[]  ReciprocalOutMin=[]  ReciprocalOutMax=[]  DivideOutMin=[]  DivideOutMax=[]  TunerSelectOption=Transfer Function Based (PID Tuner App)
  cfblk13 : DiscreteFir
  cfblk14 : Delay  ShowEnablePort=on
      settings: InputPortMap=u0,e6
  cfblk15 : simulink/Discrete/Tapped Delay  vinit=0.0  samptime=-1  NumDelays=1  DelayOrder=Oldest  includeCurrent=off
  cfblk18 : Delay
  cfblk19 : Delay
  cfblk3 : simulink/Discrete/Difference  ICPrevInput=0.0  OutMin=[]  OutMax=[]  OutDataTypeStr=Inherit: Inherit via back propagation  OutDataType=fixdt(1, 16)  OutScaling=2^-10  DoSatur=off
  cfblk4 : simulink/Discrete/Transfer Fcn Real Zero  ZeroZ=0.75  ICPrevInput=0.0  DoSatur=off
      settings: SourceProductName=Simulink  SourceProductBaseCode=SL
  cfblk5 : simulink/Discrete/Difference  ICPrevInput=0.0  OutMin=[]  OutMax=[]  OutDataTypeStr=Inherit: Inherit via back propagation  OutDataType=fixdt(1, 16)  OutScaling=2^-10  DoSatur=off
  cfblk6 : Delay  DelayLengthSource=Input port
      settings: InputPortMap=u0,p1
  cfblk7 : DiscreteStateSpace  SampleTime=-1
  cfblk8 : simulink/Discrete/Transfer Fcn Lead or Lag  PoleZ=0.95  ZeroZ=0.75  ICPrevOutput=0.0  ICPrevInput=0.0  DoSatur=off
      settings: SourceProductName=Simulink  SourceProductBaseCode=SL
  cfblk9 : DiscreteFir
  cyemi_{99..116} (18 alike) : DataTypeConversion  OutDataTypeStr=double
  cfblk2 : Outport
  cfblk17 : Outport  Port=2
  wires:
  cfblk15/1 -> cfblk17/1
  cfblk7/1 -> cyemi_100/1, cyemi_103/1
  cfblk9/1 -> cfblk2/1
  cfblk3/1 -> cyemi_112/1, cyemi_116/1
  cfblk8/1 -> cyemi_105/1, cyemi_107/1
  cyemi_99/1 -> cfblk10/1
  cfblk16/1 -> cyemi_99/1
  cyemi_100/1 -> cfblk11/1
  cyemi_101/1 -> cfblk12/1
  cfblk5/1 -> cyemi_101/1
  cyemi_102/1 -> cfblk12/2
  cfblk18/1 -> cyemi_102/1
  cyemi_103/1 -> cfblk13/1
  cyemi_104/1 -> cfblk14/1
  cfblk10/1 -> cyemi_104/1
  cyemi_105/1 -> cfblk14/2
  cyemi_106/1 -> cfblk15/1
  cfblk14/1 -> cyemi_106/1
  cyemi_107/1 -> cfblk18/1
  cyemi_108/1 -> cfblk19/1
  cfblk13/1 -> cyemi_108/1
  cyemi_109/1 -> cfblk3/1
  cfblk11/1 -> cyemi_109/1
  cyemi_110/1 -> cfblk4/1
  cfblk1/1 -> cyemi_110/1
  cyemi_111/1 -> cfblk5/1
  cfblk6/1 -> cyemi_111/1
  cyemi_112/1 -> cfblk6/1
  cyemi_113/1 -> cfblk6/2
  cfblk4/1 -> cyemi_113/1
  cyemi_114/1 -> cfblk7/1
  cfblk19/1 -> cyemi_114/1
  cyemi_115/1 -> cfblk8/1
  cfblk12/1 -> cyemi_115/1
  cyemi_116/1 -> cfblk9/1

== system sampleModel2432_pp/cfblk197/cfblk18 ==
  cfblk1 : Inport
  cfblk9 : Inport  Port=2
  cfblk10 : Inport  Port=3
  Action Port : ActionPort  ActionType=else
  cfblk3 : Delay
  cfblk4 : Delay
  cfblk5 : DiscreteZeroPole  Poles=[0 0.5]  Gain=1  SampleTime=-1
  cfblk6 : simulink/Continuous/PID Controller  Controller=PID  TimeDomain=Discrete-time  SampleTime=-1  IntegratorMethod=Forward Euler  FilterMethod=Forward Euler  Form=Parallel  UseFilter=on  ControllerParametersSource=internal  P=1  I=1  D=0  N=100  InitialConditionSource=internal  InitialConditionForIntegrator=0  InitialConditionForFilter=0  ExternalReset=none  LimitOutput=off  UpperSaturationLimit=inf  LowerSaturationLimit=-inf  LinearizeAsGain=off  AntiWindupMode=none  Kb=1  TrackingMode=off  Kt=1  PParamMin=[]  PParamMax=[]  IParamMin=[]  IParamMax=[]  DParamMin=[]  DParamMax=[]  NParamMin=[]  NParamMax=[]  KbParamMin=[]  KbParamMax=[]  KtParamMin=[]  KtParamMax=[]  POutMin=[]  POutMax=[]  IOutMin=[]  IOutMax=[]  DOutMin=[]  DOutMax=[]  NOutMin=[]  NOutMax=[]  KbOutMin=[]  KbOutMax=[]  KtOutMin=[]  KtOutMax=[]  IntegratorOutMin=[]  IntegratorOutMax=[]  FilterOutMin=[]  FilterOutMax=[]  SumOutMin=[]  SumOutMax=[]  SumI1OutMin=[]  SumI1OutMax=[]  SumI2OutMin=[]  SumI2OutMax=[]  SumI3OutMin=[]  SumI3OutMax=[]  SumDOutMin=[]  SumDOutMax=[]  SaturationOutMin=[]  SaturationOutMax=[]  IntegratorContinuousStateAttributes=''  IntegratorStateMustResolveToSignalObject=off  IntegratorRTWStateStorageClass=Auto  FilterContinuousStateAttributes=''  FilterStateMustResolveToSignalObject=off  FilterRTWStateStorageClass=Auto  DifferentiatorICPrevScaledInput=0  DifferentiatorOutMin=[]  DifferentiatorOutMax=[]  FilterDiffOutCoefMin=[]  FilterDiffOutCoefMax=[]  SumDenOutMin=[]  SumDenOutMax=[]  SumNumOutMin=[]  SumNumOutMax=[]  ReciprocalOutMin=[]  ReciprocalOutMax=[]  DivideOutMin=[]  DivideOutMax=[]  TunerSelectOption=Transfer Function Based (PID Tuner App)
  cfblk7 : simulink/Discrete/Transfer Fcn Real Zero  ZeroZ=0.75  ICPrevInput=0.0  DoSatur=off
      settings: SourceProductName=Simulink  SourceProductBaseCode=SL
  cfblk8 : DiscreteFilter
  cyemi_{120..125} (6 alike) : DataTypeConversion  OutDataTypeStr=double
  cfblk2 : Outport
  cfblk11 : Outport  Port=2
  wires:
  cfblk8/1 -> cfblk11/1
  cfblk1/1 -> cfblk2/1
  cyemi_120/1 -> cfblk3/1
  cfblk4/1 -> cyemi_120/1
  cyemi_121/1 -> cfblk4/1
  cfblk6/1 -> cyemi_121/1
  cyemi_122/1 -> cfblk5/1
  cfblk9/1 -> cyemi_122/1
  cyemi_123/1 -> cfblk6/1
  cfblk10/1 -> cyemi_123/1
  cyemi_124/1 -> cfblk7/1
  cfblk3/1 -> cyemi_124/1
  cyemi_125/1 -> cfblk8/1
  cfblk7/1 -> cyemi_125/1

== system sampleModel2432_pp/cfblk198/cfblk13 ==
  cfblk1 : Inport
  cfblk13 : Inport  Port=2
  Action Port : ActionPort  ActionType=then
  cfblk10 : simulink/Discrete/Transfer Fcn Real Zero  ZeroZ=0.75  ICPrevInput=0.0  DoSatur=off
      settings: SourceProductName=Simulink  SourceProductBaseCode=SL
  cfblk11 : DiscreteFilter
  cfblk12 : simulink/Discrete/Transfer Fcn Lead or Lag  PoleZ=0.95  ZeroZ=0.75  ICPrevOutput=0.0  ICPrevInput=0.0  DoSatur=off
      settings: SourceProductName=Simulink  SourceProductBaseCode=SL
  cfblk17 : Delay
  cfblk3 : Delay  DelayLengthSource=Input port
      settings: InputPortMap=u0,p1
  cfblk4 : simulink/Discrete/Tapped Delay  vinit=0.0  samptime=-1  NumDelays=1  DelayOrder=Oldest  includeCurrent=off
  cfblk5 : DiscreteIntegrator  SampleTime=-1  ICPrevOutput=DiscIntNeverNeededParam  ICPrevScaledInput=DiscIntNeverNeededParam
  cfblk6 : simulink/Continuous/PID Controller (2DOF)  Controller=PID  TimeDomain=Discrete-time  SampleTime=-1  IntegratorMethod=Forward Euler  FilterMethod=Forward Euler  Form=Parallel  UseFilter=on  ControllerParametersSource=internal  P=1  I=1  D=0  N=100  b=1  c=1  InitialConditionSource=internal  InitialConditionForIntegrator=0  InitialConditionForFilter=0  ExternalReset=none  LimitOutput=off  UpperSaturationLimit=inf  LowerSaturationLimit=-inf  LinearizeAsGain=off  AntiWindupMode=none  Kb=1  TrackingMode=off  Kt=1  PParamMin=[]  PParamMax=[]  IParamMin=[]  IParamMax=[]  DParamMin=[]  DParamMax=[]  NParamMin=[]  NParamMax=[]  bParamMin=[]  bParamMax=[]  cParamMin=[]  cParamMax=[]  KbParamMin=[]  KbParamMax=[]  KtParamMin=[]  KtParamMax=[]  POutMin=[]  POutMax=[]  IOutMin=[]  IOutMax=[]  DOutMin=[]  DOutMax=[]  NOutMin=[]  NOutMax=[]  bOutMin=[]  bOutMax=[]  cOutMin=[]  cOutMax=[]  KbOutMin=[]  KbOutMax=[]  KtOutMin=[]  KtOutMax=[]  IntegratorOutMin=[]  IntegratorOutMax=[]  FilterOutMin=[]  FilterOutMax=[]  SumOutMin=[]  SumOutMax=[]  Sum1OutMin=[]  Sum1OutMax=[]  Sum2OutMin=[]  Sum2OutMax=[]  Sum3OutMin=[]  Sum3OutMax=[]  SumI1OutMin=[]  SumI1OutMax=[]  SumI2OutMin=[]  SumI2OutMax=[]  SumI3OutMin=[]  SumI3OutMax=[]  SumDOutMin=[]  SumDOutMax=[]  SaturationOutMin=[]  SaturationOutMax=[]  IntegratorContinuousStateAttributes=''  IntegratorStateMustResolveToSignalObject=off  IntegratorRTWStateStorageClass=Auto  FilterContinuousStateAttributes=''  FilterStateMustResolveToSignalObject=off  FilterRTWStateStorageClass=Auto  DifferentiatorICPrevScaledInput=0  DifferentiatorOutMin=[]  DifferentiatorOutMax=[]  FilterDiffOutCoefMin=[]  FilterDiffOutCoefMax=[]  SumDenOutMin=[]  SumDenOutMax=[]  SumNumOutMin=[]  SumNumOutMax=[]  ReciprocalOutMin=[]  ReciprocalOutMax=[]  DivideOutMin=[]  DivideOutMax=[]  TunerSelectOption=Transfer Function Based (PID Tuner App)
  cfblk7 : Delay  DelayLengthSource=Input port
      settings: InputPortMap=u0,p1
  cfblk8 : Delay  DelayLengthSource=Input port
      settings: InputPortMap=u0,p1
  cfblk9 : DiscreteFir
  cyemi_{147..161} (15 alike) : DataTypeConversion  OutDataTypeStr=double
  cfblk2 : Outport
  cfblk14 : Outport  Port=2
  cfblk15 : Outport  Port=3
  cfblk16 : Outport  Port=4
  wires:
  cfblk1/1 -> cyemi_147/1, cyemi_155/1, cyemi_158/1
  cfblk4/1 -> cfblk2/1, cyemi_156/1
  cfblk12/1 -> cyemi_154/1, cyemi_161/1
  cfblk13/1 -> cfblk14/1
  cfblk6/1 -> cfblk15/1, cyemi_150/1, cyemi_159/1
  cfblk8/1 -> cfblk16/1
  cyemi_147/1 -> cfblk10/1
  cyemi_148/1 -> cfblk11/1
  cfblk10/1 -> cyemi_148/1
  cyemi_149/1 -> cfblk12/1
  cfblk11/1 -> cyemi_149/1
  cyemi_150/1 -> cfblk17/1
  cyemi_151/1 -> cfblk3/1
  cfblk9/1 -> cyemi_151/1
  cyemi_152/1 -> cfblk3/2
  cfblk17/1 -> cyemi_152/1
  cyemi_153/1 -> cfblk4/1
  cfblk3/1 -> cyemi_153/1
  cyemi_154/1 -> cfblk5/1
  cyemi_155/1 -> cfblk6/1
  cyemi_156/1 -> cfblk6/2
  cyemi_157/1 -> cfblk7/1
  cfblk5/1 -> cyemi_157/1
  cyemi_158/1 -> cfblk7/2
  cyemi_159/1 -> cfblk8/1
  cyemi_160/1 -> cfblk8/2
  cfblk7/1 -> cyemi_160/1
  cyemi_161/1 -> cfblk9/1
